simulink model "trail2"  (R2024a)
settings: Solver=VariableStepAuto  StartTime=0.0  StopTime=10.0  RelTol=1e-3
settings Model: Creator=DELL  LastModifiedBy=DELL

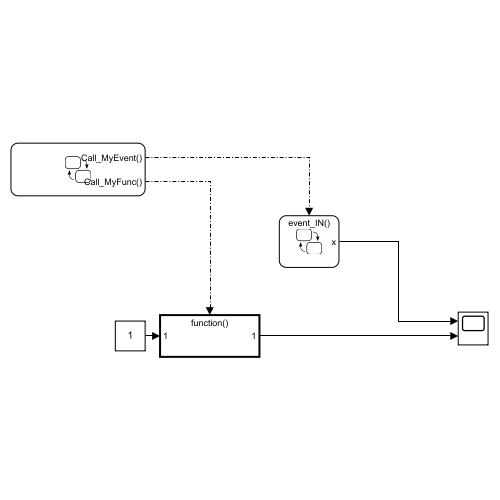
[thumbnail: Simulink's stored preview of the top-level diagram]
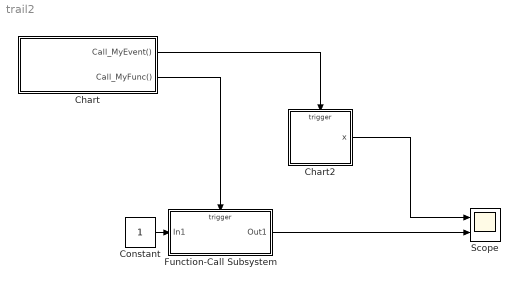
== system trail2 ==
  Chart : Stateflow chart  TreatAsAtomicUnit=on
  Chart2 : Stateflow chart  TreatAsAtomicUnit=on
  Constant : Constant
  Function-Call Subsystem : Subsystem  TreatAsAtomicUnit=on
  Scope : Scope  NumInputPorts=2
  wires:
  Chart/2(Call_MyFunc()) -> Function-Call Subsystem/Trigger
  Constant/1 -> Function-Call Subsystem/1(In1)
  Function-Call Subsystem/1(Out1) -> Scope/2
  Chart/1(Call_MyEvent()) -> Chart2/Trigger
  Chart2/1(x) -> Scope/1

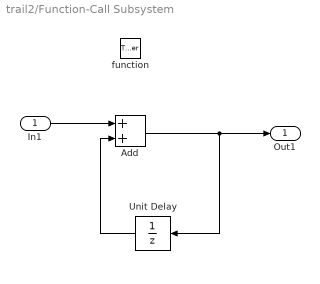
== system trail2/Function-Call Subsystem ==
  In1 : Inport
  function : TriggerPort  TriggerType=function-call  VariantControl=(inherit)
  Add : Sum
  Unit Delay : UnitDelay  SampleTime=-1  HasFrameUpgradeWarning=on
  Out1 : Outport
  wires:
  In1/1 -> Add/1
  Unit Delay/1 -> Add/2
  Add/1 -> Unit Delay/1, Out1/1

== stateflow chart trail2/Chart2 ==
  state State_A
    en:
    x=3;
  state State_B
    en:
    x=6;
  (default) -> State_A
  State_A -> State_B : event_IN
  State_B -> State_A : event_IN
  data: x output
  events: event_IN input FUNCTION_CALL_EVENT

== stateflow chart trail2/Chart ==
  state State_A [parallel]
    settings: executionOrder=1
    state A
    A -> A : after(1,sec)/{Call_MyFunc}
  state State_B [parallel]
    settings: executionOrder=2
    state B
    B -> B : after(1,sec)/{Call_MyEvent}
  (default) -> A
  events: Call_MyEvent output FUNCTION_CALL_EVENT; Call_MyFunc output FUNCTION_CALL_EVENT
